simulink library "InputDeviceHandler"  (R2016b)
settings: Solver=VariableStepAuto  StartTime=0.0  StopTime=10.0  RelTol=1e-3
undefined symbols (not defined in the file or in its folder): EthercatDeviceError
libraries: TimestampChecker x1
settings Model: Creator=Nathan  LastModifiedBy=MARCH

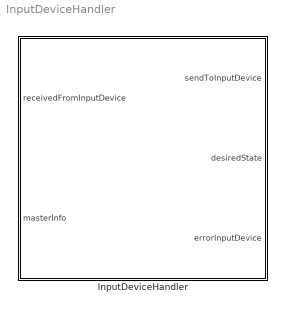
== system InputDeviceHandler ==
  InputDeviceHandler : Subsystem

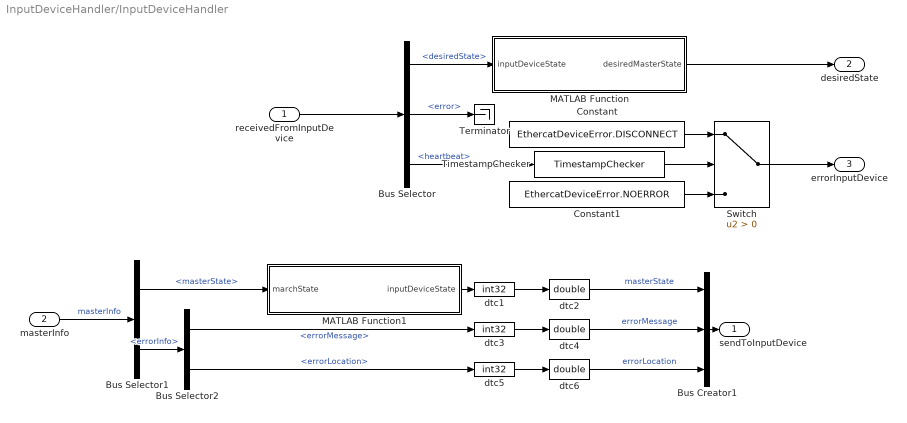
== system InputDeviceHandler/InputDeviceHandler ==
  receivedFromInputDevice : Inport  OutDataTypeStr=Bus: EtherCATReceivedFromInputDevice  BusOutputAsStruct=on
  masterInfo : Inport  Port=2
  Bus Creator1 : BusCreator  Inputs=3  OutDataTypeStr=Bus: EtherCATSendToInputDevice  NonVirtualBus=on
  Bus Selector : BusSelector  OutputSignals=desiredState,error,heartbeat
  Bus Selector1 : BusSelector  OutputSignals=masterState,errorInfo
  Bus Selector2 : BusSelector  OutputSignals=errorMessage,errorLocation
  Constant : Constant  Value=EthercatDeviceError.DISCONNECT
  Constant1 : Constant  Value=EthercatDeviceError.NOERROR
  MATLAB Function : MATLAB Function  TreatAsAtomicUnit=on
  MATLAB Function1 : MATLAB Function  TreatAsAtomicUnit=on
  Switch : Switch  Criteria=u2 > Threshold
  Terminator : Terminator
  TimestampChecker : TimestampChecker/TimestampChecker
  dtc1 : DataTypeConversion  OutDataTypeStr=int32
  dtc2 : DataTypeConversion  OutDataTypeStr=double
  dtc3 : DataTypeConversion  OutDataTypeStr=int32
  dtc4 : DataTypeConversion  OutDataTypeStr=double
  dtc5 : DataTypeConversion  OutDataTypeStr=int32
  dtc6 : DataTypeConversion  OutDataTypeStr=double
  sendToInputDevice : Outport  OutDataTypeStr=Bus: EtherCATSendToInputDevice  BusOutputAsStruct=on
  desiredState : Outport  Port=2
  errorInputDevice : Outport  Port=3  OutDataTypeStr=Enum: EthercatDeviceError
  wires:
  Switch/1 -> errorInputDevice/1
  Constant1/1 -> Switch/3
  Constant/1 -> Switch/1
  TimestampChecker/1 -> Switch/2
  Bus Selector/3 -> TimestampChecker/1  "<heartbeat>"
  dtc6/1 -> Bus Creator1/3  "errorLocation"
  Bus Selector2/2 -> dtc5/1  "<errorLocation>"
  dtc5/1 -> dtc6/1
  Bus Selector1/2 -> Bus Selector2/1  "<errorInfo>"
  Bus Selector1/1 -> MATLAB Function1/1(marchState)  "<masterState>"
  Bus Selector2/1 -> dtc3/1  "<errorMessage>"
  masterInfo/1 -> Bus Selector1/1  "masterInfo"
  MATLAB Function1/1(inputDeviceState) -> dtc1/1
  dtc4/1 -> Bus Creator1/2  "errorMessage"
  dtc3/1 -> dtc4/1
  dtc2/1 -> Bus Creator1/1  "masterState"
  dtc1/1 -> dtc2/1
  MATLAB Function/1(desiredMasterState) -> desiredState/1
  Bus Selector/1 -> MATLAB Function/1(inputDeviceState)  "<desiredState>"
  receivedFromInputDevice/1 -> Bus Selector/1
  Bus Creator1/1 -> sendToInputDevice/1
  Bus Selector/2 -> Terminator/1  "<error>"

== matlab function InputDeviceHandler/MATLAB Function ==
  data: inputDeviceState input; desiredMasterState output
function desiredMasterState = getDesiredMasterState(inputDeviceState)
%% Translates received inputDeviceState to desired ExoskeletonState
% Copy of input device source code:
%#define SIT 1
%#define STAND 2
%#define WALK 3
%#define STONES 4
%#define STAIRS_UP 5
%#define STAIRS_DOWN 6
%#define SLOPE_UP 7
%#define SLOPE_DOWN 8
%#define MANUAL 9
switch(inputDeviceState)
    case 0
        desiredMasterState = ExoskeletonState.UNREACHABLE;
    case 1 %% on disconnect, this will be zero. Need to change the values in inputDevice source
        desiredMasterState = ExoskeletonState.HOLDSIT;
    case 2
        desiredMasterState = ExoskeletonState.HOLDSTAND;
    case 3
        desiredMasterState = ExoskeletonState.CONTINUOUSGAIT;
    case 4
        desiredMasterState = ExoskeletonState.SHUTTING_DOWN;
    case 5
        desiredMasterState = ExoskeletonState.STAIRSUP; %% only one stairs currently
    case 6
        desiredMasterState = ExoskeletonState.STAIRSDOWN;
    case 7
        desiredMasterState = ExoskeletonState.SLOPE; %% only one slope currently
    case 8
        desiredMasterState = ExoskeletonState.SLOPE;
    case 9
        desiredMasterState = ExoskeletonState.MANUAL;
    otherwise
        desiredMasterState = ExoskeletonState.FULLMANUAL;
end
end

== matlab function InputDeviceHandler/MATLAB Function1 ==
  data: marchState input; inputDeviceState output
function inputDeviceState = getInputDeviceState(marchState)

switch(marchState)
    case ExoskeletonState.HOLDSIT %% on disconnect, this will be zero. Need to change the values in inputDevice source
         inputDeviceState = 1;
    case ExoskeletonState.HOLDSTAND
         inputDeviceState = 2;
    case ExoskeletonState.CONTINUOUSGAIT
         inputDeviceState = 3;
    case ExoskeletonState.STONES
         inputDeviceState = 4;
    case ExoskeletonState.STAIRSUP %%No difference between up and down atm 
         inputDeviceState = 5;
    case ExoskeletonState.STAIRSDOWN %%No difference between up and down atm 
         inputDeviceState = 6;
    case ExoskeletonState.SLOPE %%No difference between up and down atm 
         inputDeviceState = 8;
    case ExoskeletonState.MANUAL
         inputDeviceState = 9;
    case ExoskeletonState.FULLMANUAL
         inputDeviceState = 9;
    otherwise
         inputDeviceState = 20;
end
end
